simulink model "Simulink_IFT_MODEL"  (R2025a)
settings: Solver=FixedStepAuto  StartTime=0.0  StopTime=60  FixedStep=1e-5  RelTol=1e-3
model workspace (MAT data in the model file):
  Amp_1 = 1
  Amp_2 = -1
  flag = 0
  r = 0.006
undefined symbols (not defined in the file): a, a1, b, b1, DiscIntNeverNeededParam, dspblkCoreblockFVToolHelper, gcbh, Kp, Newton, Raphson, Ti
settings Model: Creator=enash  LastModifiedBy=Student
settings DataIOCC: SignalLogging=off  DSMLogging=off

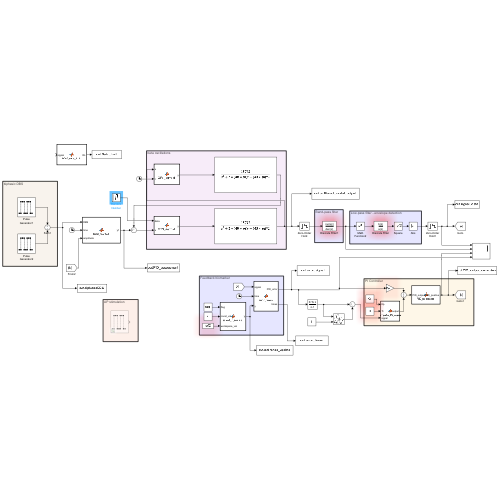
[thumbnail: Simulink's stored preview of the top-level diagram]
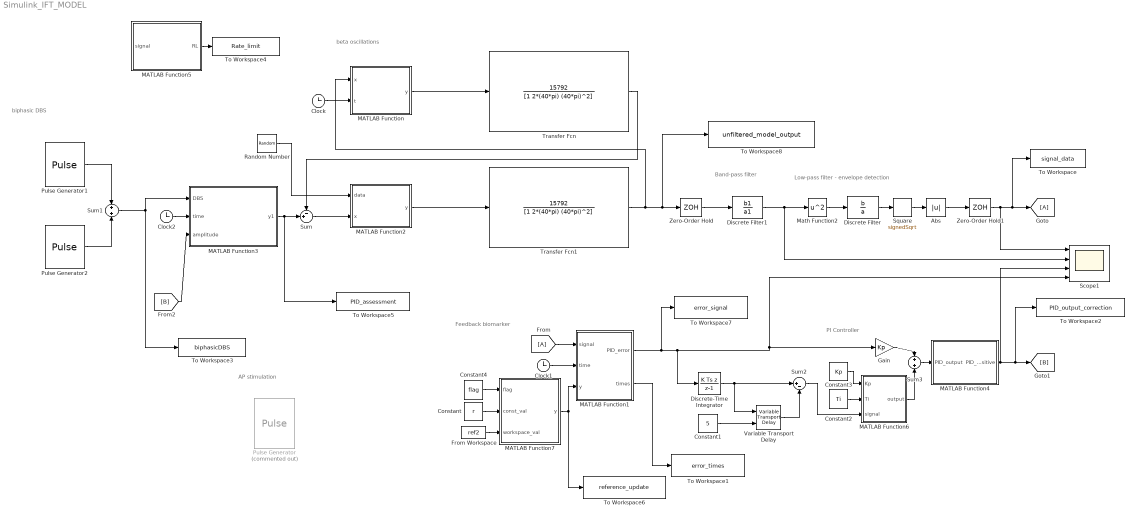
== system Simulink_IFT_MODEL ==
  note: Feedback biomarker
  note: AP stimulation
  note: biphasic DBS
  note: beta oscillations
  note: Low-pass filter - envelope detection
  note: PI Controller
  note: Band-pass filter
  Abs : Abs  SaturateOnIntegerOverflow=off
  Clock : Clock
      settings: Decimation=20
  Clock1 : Clock
      settings: Decimation=20
  Clock2 : Clock
      settings: Decimation=20
  Constant : Constant  Value=r
  Constant1 : Constant  Value=5
  Constant2 : Constant  Value=Ti
  Constant3 : Constant  Value=Kp
  Constant4 : Constant  Value=flag
  Discrete Filter : DiscreteFilter  LoadFcn=dspblkCoreblockFVToolHelper(gcbh,'load');  Numerator=b  Denominator=a
      settings: CopyFcn=dspblkCoreblockFVToolHelper(gcbh,'copy');  DeleteFcn=dspblkCoreblockFVToolHelper(gcbh,'close');  ModelCloseFcn=dspblkCoreblockFVToolHelper(gcbh,'close');  PreSaveFcn=dspblkCoreblockFVToolHelper(gcbh,'presave');  PostSaveFcn=dspblkCoreblockFVToolHelper(gcbh,'postsave');  CloseFcn=dspblkCoreblockFVToolHelper(gcbh,'close');
  Discrete Filter1 : DiscreteFilter  LoadFcn=dspblkCoreblockFVToolHelper(gcbh,'load');  Numerator=b1  Denominator=a1
      settings: CopyFcn=dspblkCoreblockFVToolHelper(gcbh,'copy');  DeleteFcn=dspblkCoreblockFVToolHelper(gcbh,'close');  ModelCloseFcn=dspblkCoreblockFVToolHelper(gcbh,'close');  PreSaveFcn=dspblkCoreblockFVToolHelper(gcbh,'presave');  PostSaveFcn=dspblkCoreblockFVToolHelper(gcbh,'postsave');  CloseFcn=dspblkCoreblockFVToolHelper(gcbh,'close');
  Discrete-Time Integrator : DiscreteIntegrator  IntegratorMethod=Integration: Backward Euler  SampleTime=-1  ICPrevOutput=DiscIntNeverNeededParam  ICPrevScaledInput=DiscIntNeverNeededParam
  From : From
  From Workspace : FromWorkspace  VariableName=ref2
  Gain : Gain  Gain=Kp
  Goto : Goto
  MATLAB Function : MATLAB Function  TreatAsAtomicUnit=on
  MATLAB Function1 : MATLAB Function  TreatAsAtomicUnit=on
  MATLAB Function2 : MATLAB Function  TreatAsAtomicUnit=on
  MATLAB Function3 : MATLAB Function  TreatAsAtomicUnit=on
  MATLAB Function4 : MATLAB Function  TreatAsAtomicUnit=on
  MATLAB Function5 : MATLAB Function  TreatAsAtomicUnit=on
  MATLAB Function6 : MATLAB Function  TreatAsAtomicUnit=on
  MATLAB Function7 : MATLAB Function  TreatAsAtomicUnit=on
  Math Function2 : Math  Operator=square
  Pulse Generator : DiscretePulseGenerator  Commented=on  Amplitude=0.1  Period=2e6  PulseWidth=2e2  SampleTime=1e-5
  Pulse Generator1 : DiscretePulseGenerator  Amplitude=Amp_1  Period=770  PulseWidth=50  SampleTime=1e-5
  Pulse Generator2 : DiscretePulseGenerator  Amplitude=Amp_2  Period=770  PulseWidth=50  PhaseDelay=10  SampleTime=1e-5
  Random Number : RandomNumber  Variance=1e-6  SampleTime=1e-5
  Scope1 : Scope  NumInputPorts=4
      settings: ActiveDisplayYMinimum=-0.002  ActiveDisplayYMaximum=0.01797
  "Square " : Sqrt  Operator=signedSqrt  AlgorithmType=Newton-Raphson
  Sum : Sum  Inputs=-+|
  Sum1 : Sum  Inputs=+|+
  Sum2 : Sum  Inputs=|+-
  Sum3 : Sum  Inputs=+|+
  To Workspace : ToWorkspace  VariableName=signal_data  SampleTime=-1
  To Workspace1 : ToWorkspace  VariableName=error_times  SampleTime=-1
  To Workspace2 : ToWorkspace  VariableName=PID_output_correction  SampleTime=-1
  To Workspace3 : ToWorkspace  VariableName=biphasicDBS  SampleTime=-1
  To Workspace4 : ToWorkspace  VariableName=Rate_limit  SampleTime=-1
  To Workspace5 : ToWorkspace  VariableName=PID_assessment  SampleTime=-1
  To Workspace6 : ToWorkspace  VariableName=reference_update  SampleTime=-1
  To Workspace7 : ToWorkspace  VariableName=error_signal  SampleTime=-1
  To Workspace8 : ToWorkspace  VariableName=unfiltered_model_output  SampleTime=-1
  Transfer Fcn : TransferFcn  Numerator=[15792]  Denominator=[1 2*(40*pi) (40*pi)^2]
  Transfer Fcn1 : TransferFcn  Numerator=[15792]  Denominator=[1 2*(40*pi) (40*pi)^2]
  Variable Transport Delay : VariableTransportDelay  MaximumDelay=10  MaximumPoints=1000448  FixedBuffer=on
  Zero-Order Hold : ZeroOrderHold  SampleTime=1e-2
  Zero-Order Hold1 : ZeroOrderHold  SampleTime=1e-5
  wires:
  MATLAB Function/1(y) -> Transfer Fcn/1
  MATLAB Function2/1(y) -> Transfer Fcn1/1
  Transfer Fcn/1 -> Sum/1
  Sum/1 -> MATLAB Function2/2(x)
  Clock/1 -> MATLAB Function/2(t)
  Pulse Generator2/1 -> Sum1/2
  Pulse Generator1/1 -> Sum1/1
  From/1 -> MATLAB Function1/1(signal)
  Sum1/1 -> MATLAB Function3/1(DBS), To Workspace3/1
  MATLAB Function1/2(times) -> To Workspace1/1
  Sum3/1 -> MATLAB Function4/1(PID_output)
  MATLAB Function3/1(y1) -> To Workspace5/1, Sum/2
  [B] -> MATLAB Function3/3(amplitude)
  MATLAB Function5/1(RL) -> To Workspace4/1
  Clock1/1 -> MATLAB Function1/2(time)
  Discrete Filter/1 -> "Square "/1
  MATLAB Function1/1(PID_error) -> Gain/1, Scope1/4, Discrete-Time Integrator/1, To Workspace7/1
  Random Number/1 -> MATLAB Function2/1(data)
  Math Function2/1 -> Discrete Filter/1
  "Square "/1 -> Abs/1
  Transfer Fcn1/1 -> Zero-Order Hold/1, To Workspace8/1, MATLAB Function/1(x)
  Clock2/1 -> MATLAB Function3/2(time)
  Zero-Order Hold/1 -> Discrete Filter1/1
  Discrete Filter1/1 -> Math Function2/1, Scope1/2
  Abs/1 -> Zero-Order Hold1/1
  Discrete-Time Integrator/1 -> Variable Transport Delay/1, Sum2/1
  Variable Transport Delay/1 -> Sum2/2
  MATLAB Function6/1(output) -> Sum3/2
  Gain/1 -> Sum3/1
  Constant1/1 -> Variable Transport Delay/2
  Sum2/1 -> MATLAB Function6/3(signal)
  Constant3/1 -> MATLAB Function6/1(Kp)
  Constant2/1 -> MATLAB Function6/2(Ti)
  Zero-Order Hold1/1 -> Goto/1, To Workspace/1, Scope1/1
  From Workspace/1 -> MATLAB Function7/3(workspace_val)
  MATLAB Function7/1(y) -> MATLAB Function1/3(y), To Workspace6/1
  Constant/1 -> MATLAB Function7/2(const_val)
  Constant4/1 -> MATLAB Function7/1(flag)
  MATLAB Function4/1(PID_positive) -> Scope1/3, To Workspace2/1, [B]

== matlab function Simulink_IFT_MODEL/MATLAB Function1 ==
  data: PID_error output; signal input; times output; time input; y input
function [PID_error, times] = error_times(signal, time, y)

% Threshold
threshold = 1e-3;

% Initialize times array
times = zeros(1, length(signal));

for i = 1:length(signal)
    if signal(i) > threshold
        times(i) = time(i);
    else
        times(i) = 0;
    end
end

%% Calculating controller error
% b_target = 0.0051; % 20-th percentile of beta ARV with no DBS

% b_target = r; % 5% of the maximum value beta oscillations for no DBS
% b_target = max(0.01 * signal, 1e-3); % stimulation threshold set to 0.1% of the beta ARV to obtain a high-level of suppression

%% Calculating controller error
PID_error = zeros(1, length(signal)); % Initialize PID_error array

% first try to normalise the signal

if time > 20
    for i = 1:length(signal)
        if isscalar(y)
            PID_error(i) = (signal(i) - y(i))/y(i);
        elseif y(i) == 0
            PID_error(i) = (signal(i) - y(i));
        else
            PID_error(i) = (signal(i) - y(i))/y(i);
        end
    end
else 
    PID_error = 0;
end

end

== matlab function Simulink_IFT_MODEL/MATLAB Function ==
  settings: updateMethod=DISCRETE
  data: x input; y output; t input
function y = GPe_sigmoid(x,t)

% % h is the sharpness parameter of the GPe sigmoid function
% if t >= 0 && t <= 20
%     h = 1.0;
% elseif t >= 1.5 && t <= 2.0
%     h = 1.0;
% elseif t >= 3.0 && t <= 5.0
%     h = 1.0;
% elseif t >= 8 && t<= 15
%     h = 1.0;
% elseif t >= 18 && t <= 40
%     h = 1.0;
% elseif t >= 43 && t <= 50
%     h = 1.0;
% else 
%     h = 0.1;
% end

% dopamine levels
% Define the range of possible values
values = 0.099:0.001:0.1;



% 20 - 35 & 35 - 40
% 
% if t >= 20 && t < 22
%     h = 0.11;
% elseif t >= 22 && t < 24
%     h = 1.0;
% elseif t >= 40 && t <= 44
%     h = 0.11;
% elseif t >= 44 && t < 46
%     h = 1.0;
% elseif t >= 65 && t <= 68
%     h = 0.11;
% elseif t >= 68 && t < 70
%     h = 1.0;
% elseif t >= 90 && t <= 92
%     h = 0.11;
% elseif t >= 92 && t < 100
%     h = 1.0;
% else
%     % Randomly select one value from the range
%     h = values(randi(length(values)));
% end

% if t >= 20 * 0.375 && t < 22 * 0.375
%     h = 0.11;
% elseif t >= 22 * 0.375 && t < 24 * 0.375
%     h = 1.0;
% elseif t >= 40 * 0.375 && t <= 44 * 0.375
%     h = 0.11;
% elseif t >= 44 * 0.375 && t < 46 * 0.375
%     h = 1.0;
% elseif t >= 65 * 0.375 && t <= 68 * 0.375
%     h = 0.11;
% elseif t >= 68 * 0.375 && t < 70 * 0.375
%     h = 1.0;
% elseif t >= 90 * 0.375 && t <= 92 * 0.375
%     h = 0.11;
% elseif t >= 92 * 0.375 && t < 100 * 0.375
%     h = 1.0;
% else
%     % Randomly select one value from the range
%     h = values(randi(length(values)));
% end


% if t >= 0 && t < 2
%     h = 1.0;
% elseif t >= 20 && t <= 25
%     h = 1.0;
% else
%     h = 0.1;
% end

% t_mod = mod(t, 20);
% 
% h = 0.1 + (1-0.1).*abs((t_mod - 10)/10);

h = 0.1;


% output of GPe sigmoid function
y = (2/pi)*atan(x/h);

end

== matlab function Simulink_IFT_MODEL/MATLAB Function2 ==
  data: data input; x input; y output
function y = STN_sigmoid(data, x)

% Ensure data and x are the same length
if length(data) ~= length(x)
    error('data and x must have the same length');
end

y = zeros(1, length(x)); % Define y with known size

% dopamine levels
g = 1.0;

for i = 1:length(x)
    % output of GPe sigmoid function
    y(i) = (2/pi)*atan((data(i)+x(i))/g);
end

end

== matlab function Simulink_IFT_MODEL/MATLAB Function3 ==
  data: DBS input; time input; amplitude input; y1 output
function y1 = DBS_Control(DBS, time, amplitude)

% DBS_amp = zeros(1, length(DBS));

% %% Varying the DBS impulse on and off for different portions
% if time <= 30
%     DBS_amp = 0;
% elseif time > 30
%     DBS_amp = DBS;
% end

% % Normalize DBS waveform to have an amplitude of 1
% normalised_DBS = DBS / max(abs(DBS));

%% Implementation of PID controller output
% Element wise multiplication of DBS and Beta
for i = 1:length(amplitude)
    if amplitude == 0
        y1 = 0;
    else
        y1 = DBS.*amplitude;
    end
end



% %% Rate limiter
% Ts = 10;
% 
% % Calculate the maximum change per time step
% delta_u = RL * Ts;
% % delta_u = 2;
% 
% % Initialize output signal
% y = zeros(size(y1));  % Same size as DBS signal
% 
% % Loop through each DBS impulse value
% for i = 1:length(y1)
%     % Check if we need to ramp the DBS value
%     if y1(i) < -4.8
%         % Ramp up DBS impulse
%         new_value = y1(i) + delta_u;
%         % Ensure the value does not exceed the maximum impulse
%         y(i) = min(new_value, 5);
%     elseif y1(i) > 4.8
%         % Ramp down DBS impulse
%         new_value = y1(i) - delta_u;
%         % Ensure the value does not fall below the minimum impulse
%         y(i) = max(new_value, -5);
%     else
%         % If DBS is at the target amplitude, maintain it
%         y(i) = y1(i);
%     end
% end

end

== matlab function Simulink_IFT_MODEL/MATLAB Function4 ==
  data: PID_output input; PID_positive output
function PID_positive = PID_correction(PID_output)

% PID_norm = zeros(1, length(signal));

% base amplitudes
% base_amplitude = 0.5;

% initialise the amplitude arrays
% amplitude = zeros(1, length(signal));

PID_positive = zeros(1, length(PID_output));

% removes the negative DC offset from zero
for i = 1:length(PID_output)

    % condition for PID output to be positive only - negative portion
    % distorts the DBS amplitude
    if PID_output < 0
        PID_positive(i) = 0;
        % PID_positive(i) = -PID_output(i);
    else
        PID_positive(i) = min(PID_output(i), 5);
        % PID_positive(i) = PID_output(i);
    end
end

== matlab function Simulink_IFT_MODEL/MATLAB Function5 ==
  data: signal input; RL output
function RL = DBS_rate_limit(signal)

% Sample time
Ts = 1e-5;
Tramp = 2;

% Calculate the rate limit
RL = Ts*(5 + 5)/Tramp;

end

== matlab function Simulink_IFT_MODEL/MATLAB Function6 ==
  data: Kp input; output output; Ti input; signal input
function output = compute_Ki_signal(Kp, Ti, signal)
    % Validate inputs
    if Ti == 0 || Kp == 0
        Ki = 0; % If either Ti or Kp is zero, Ki should be zero
    else
        Ki = Kp / Ti; % Compute Ki
    end
    
    % Multiply Ki element-wise with the signal
    output = Ki * signal;
end

== matlab function Simulink_IFT_MODEL/MATLAB Function7 ==
  data: flag input; y output; const_val input; workspace_val input
function y = select_r_source(flag, const_val, workspace_val)
    if flag == 0
        y = const_val;
    else
        y = workspace_val;
    end
end
